simulink model "gm_dadda_mult"  (R2015a)
settings: Solver=ode45  StartTime=0.0  StopTime=10.0  RelTol=1e-3
settings Model: Creator=citdmath  LastModifiedBy=citdmath
settings OptimizationCC: BlockReduction=off  ConditionallyExecuteInputs=off
settings DebuggingCC: InheritedTsInSrcMsg=none

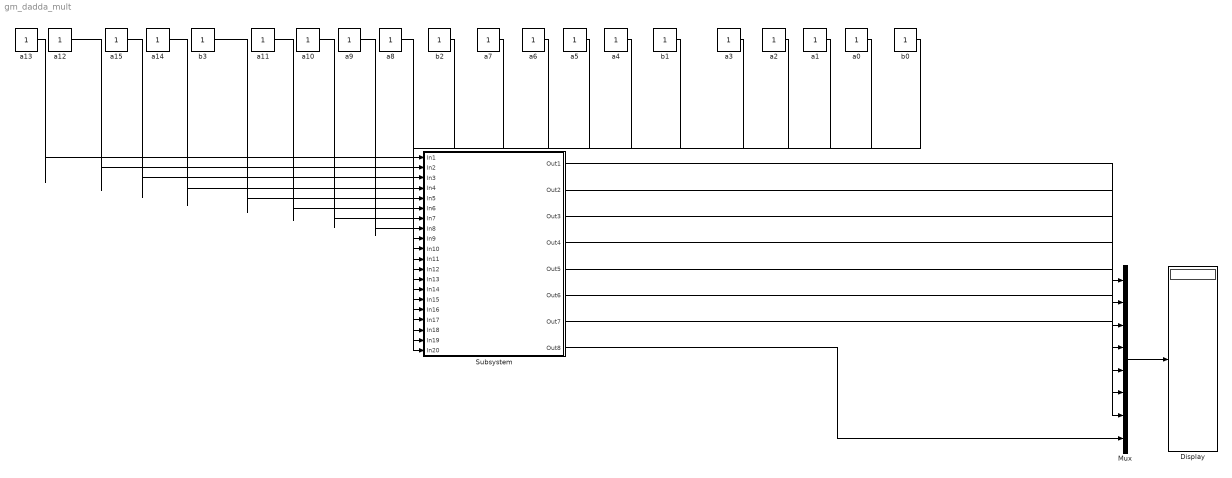
== system gm_dadda_mult ==
  Display : Display
  Mux : Mux  Inputs=8
  Subsystem : Subsystem
  a{0..15} (16 alike) : Constant
  b{0..3} (4 alike) : Constant
  wires:
  Subsystem/8(Out8) -> Mux/8
  Subsystem/7(Out7) -> Mux/7
  Subsystem/6(Out6) -> Mux/6
  Subsystem/5(Out5) -> Mux/5
  Subsystem/4(Out4) -> Mux/4
  Subsystem/3(Out3) -> Mux/3
  Subsystem/2(Out2) -> Mux/2
  Subsystem/1(Out1) -> Mux/1
  b0/1 -> Subsystem/20(In20)
  a0/1 -> Subsystem/19(In19)
  a1/1 -> Subsystem/18(In18)
  a2/1 -> Subsystem/17(In17)
  a3/1 -> Subsystem/16(In16)
  b1/1 -> Subsystem/15(In15)
  a4/1 -> Subsystem/14(In14)
  a5/1 -> Subsystem/13(In13)
  a6/1 -> Subsystem/12(In12)
  a7/1 -> Subsystem/11(In11)
  b2/1 -> Subsystem/10(In10)
  a8/1 -> Subsystem/9(In9)
  a9/1 -> Subsystem/8(In8)
  a10/1 -> Subsystem/7(In7)
  a11/1 -> Subsystem/6(In6)
  b3/1 -> Subsystem/5(In5)
  a14/1 -> Subsystem/4(In4)
  a15/1 -> Subsystem/3(In3)
  a12/1 -> Subsystem/2(In2)
  a13/1 -> Subsystem/1(In1)
  Mux/1 -> Display/1

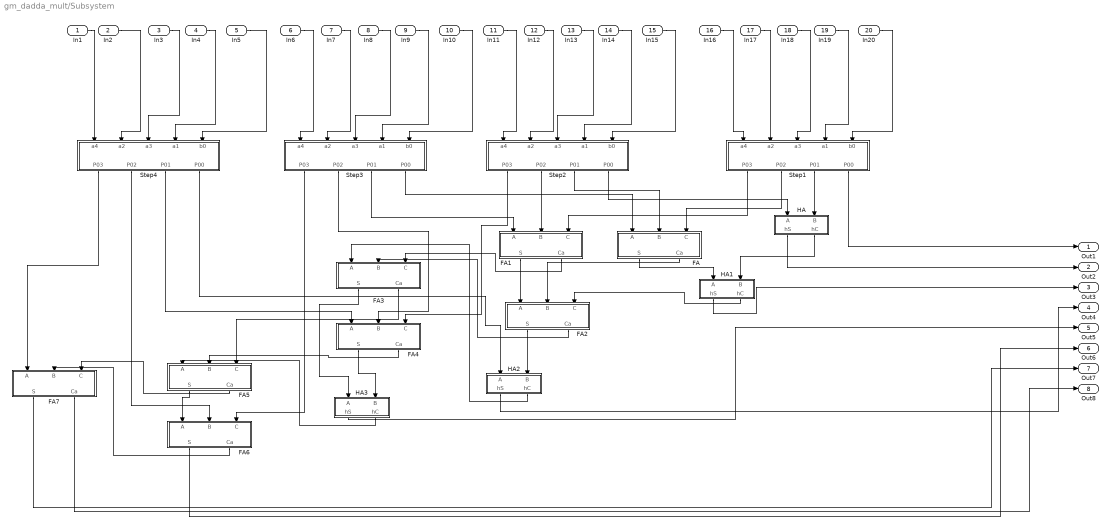
== system gm_dadda_mult/Subsystem ==
  In1 : Inport
  In2 : Inport  Port=2
  In3 : Inport  Port=3
  In4 : Inport  Port=4
  In5 : Inport  Port=5
  In6 : Inport  Port=6
  In7 : Inport  Port=7
  In8 : Inport  Port=8
  In9 : Inport  Port=9
  In10 : Inport  Port=10
  In11 : Inport  Port=11
  In12 : Inport  Port=12
  In13 : Inport  Port=13
  In14 : Inport  Port=14
  In15 : Inport  Port=15
  In16 : Inport  Port=16
  In17 : Inport  Port=17
  In18 : Inport  Port=18
  In19 : Inport  Port=19
  In20 : Inport  Port=20
  FA : Subsystem
  FA1 : Subsystem
  FA2 : Subsystem
  FA3 : Subsystem
  FA4 : Subsystem
  FA5 : Subsystem
  FA6 : Subsystem
  FA7 : Subsystem
  HA : Subsystem
  HA1 : Subsystem
  HA2 : Subsystem
  HA3 : Subsystem
  Step1 : Subsystem
  Step2 : Subsystem
  Step3 : Subsystem
  Step4 : Subsystem
  Out1 : Outport
  Out2 : Outport  Port=2
  Out3 : Outport  Port=3
  Out4 : Outport  Port=4
  Out5 : Outport  Port=5
  Out6 : Outport  Port=6
  Out7 : Outport  Port=7
  Out8 : Outport  Port=8
  wires:
  FA/2(Ca) -> FA2/2(B)
  Step3/3(P01) -> FA1/1(A)
  FA5/1(S) -> FA6/1(A)
  FA2/1(S) -> HA2/2(B)
  FA2/2(Ca) -> FA3/2(B)
  HA2/1(hS) -> Out4/1
  Step2/2(P02) -> FA1/2(B)
  Step2/1(P03) -> FA4/3(C)
  FA1/2(Ca) -> FA3/3(C)
  FA1/1(S) -> FA2/1(A)
  HA3/2(hC) -> FA5/1(A)
  FA5/2(Ca) -> FA7/3(C)
  FA4/1(S) -> HA3/2(B)
  FA7/2(Ca) -> Out8/1
  FA3/2(Ca) -> FA5/3(C)
  FA3/1(S) -> HA3/1(A)
  Step1/1(P03) -> FA1/3(C)
  Step4/4(P00) -> HA2/1(A)
  HA1/1(hS) -> Out3/1
  HA1/2(hC) -> FA2/3(C)
  FA/1(S) -> HA1/1(A)
  HA3/1(hS) -> Out5/1
  FA7/1(S) -> Out7/1
  HA/2(hC) -> HA1/2(B)
  Step4/2(P02) -> FA6/2(B)
  Step3/2(P02) -> FA4/2(B)
  Step1/4(P00) -> Out1/1
  FA4/2(Ca) -> FA5/2(B)
  FA6/2(Ca) -> FA7/2(B)
  Step2/4(P00) -> HA/1(A)
  Step3/1(P03) -> FA6/3(C)
  HA/1(hS) -> Out2/1
  Step4/3(P01) -> FA4/1(A)
  Step3/4(P00) -> FA/1(A)
  In20/1 -> Step1/5(b0)
  In1/1 -> Step4/1(a4)
  In5/1 -> Step4/5(b0)
  Step1/3(P01) -> HA/2(B)
  In2/1 -> Step4/2(a2)
  In4/1 -> Step4/4(a1)
  In3/1 -> Step4/3(a3)
  In16/1 -> Step1/1(a4)
  Step4/1(P03) -> FA7/1(A)
  In9/1 -> Step3/4(a1)
  In7/1 -> Step3/2(a2)
  In6/1 -> Step3/1(a4)
  In8/1 -> Step3/3(a3)
  In10/1 -> Step3/5(b0)
  FA6/1(S) -> Out6/1
  In18/1 -> Step1/3(a3)
  In12/1 -> Step2/2(a2)
  In13/1 -> Step2/3(a3)
  In14/1 -> Step2/4(a1)
  In15/1 -> Step2/5(b0)
  In11/1 -> Step2/1(a4)
  In17/1 -> Step1/2(a2)
  HA2/2(hC) -> FA3/1(A)
  Step2/3(P01) -> FA/2(B)
  Step1/2(P02) -> FA/3(C)
  In19/1 -> Step1/4(a1)

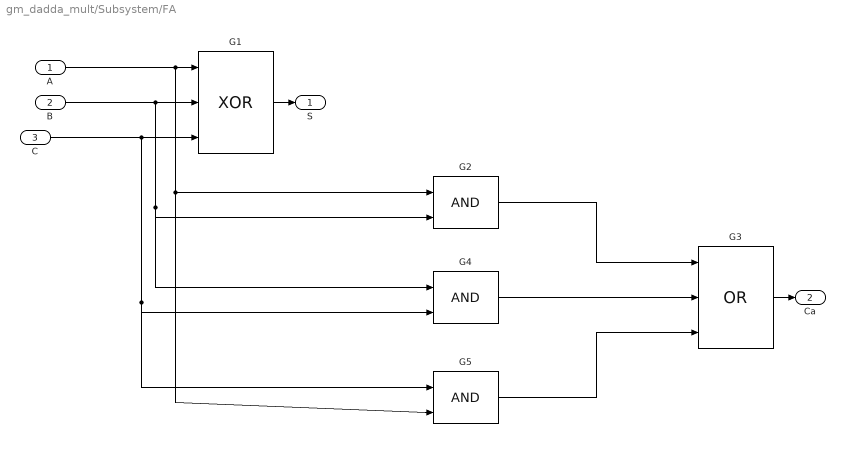
== system gm_dadda_mult/Subsystem/FA ==
  A : Inport
  B : Inport  Port=2
  C : Inport  Port=3
  G1 : Logic  Operator=XOR  Inputs=3  IconShape=distinctive  AllPortsSameDT=off  OutDataTypeStr=boolean
  G2 : Logic  IconShape=distinctive  AllPortsSameDT=off  OutDataTypeStr=boolean
  G3 : Logic  Operator=OR  Inputs=3  IconShape=distinctive  AllPortsSameDT=off  OutDataTypeStr=boolean
  G4 : Logic  IconShape=distinctive  AllPortsSameDT=off  OutDataTypeStr=boolean
  G5 : Logic  IconShape=distinctive  AllPortsSameDT=off  OutDataTypeStr=boolean
  S : Outport
  Ca : Outport  Port=2
  wires:
  G1/1 -> S/1
  G3/1 -> Ca/1
  B/1 -> G1/2, G2/2, G4/1
  G4/1 -> G3/2
  A/1 -> G1/1, G2/1, G5/2
  G2/1 -> G3/1
  C/1 -> G1/3, G4/2, G5/1
  G5/1 -> G3/3

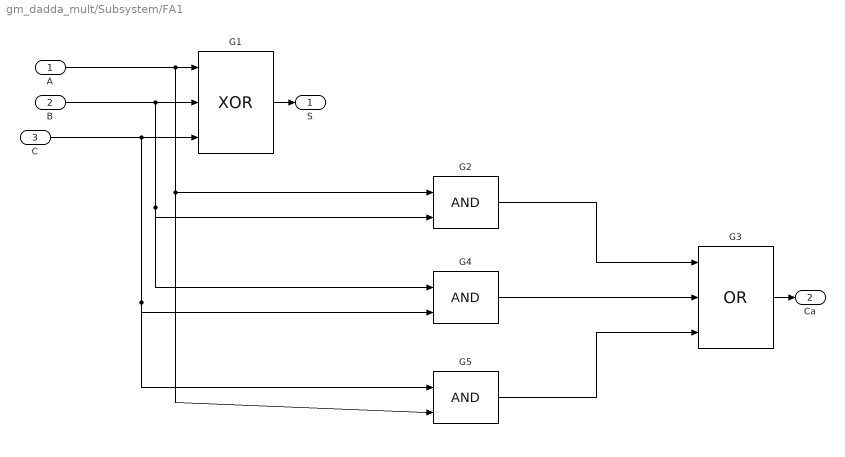
== system gm_dadda_mult/Subsystem/FA1 ==
  A : Inport
  B : Inport  Port=2
  C : Inport  Port=3
  G1 : Logic  Operator=XOR  Inputs=3  IconShape=distinctive  AllPortsSameDT=off  OutDataTypeStr=boolean
  G2 : Logic  IconShape=distinctive  AllPortsSameDT=off  OutDataTypeStr=boolean
  G3 : Logic  Operator=OR  Inputs=3  IconShape=distinctive  AllPortsSameDT=off  OutDataTypeStr=boolean
  G4 : Logic  IconShape=distinctive  AllPortsSameDT=off  OutDataTypeStr=boolean
  G5 : Logic  IconShape=distinctive  AllPortsSameDT=off  OutDataTypeStr=boolean
  S : Outport
  Ca : Outport  Port=2
  wires:
  G5/1 -> G3/3
  C/1 -> G5/1, G4/2, G1/3
  G2/1 -> G3/1
  A/1 -> G5/2, G2/1, G1/1
  G4/1 -> G3/2
  B/1 -> G4/1, G2/2, G1/2
  G3/1 -> Ca/1
  G1/1 -> S/1

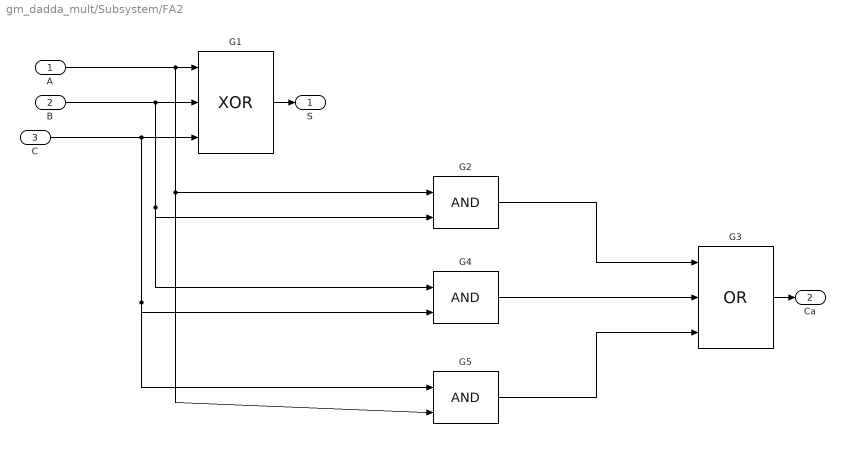
== system gm_dadda_mult/Subsystem/FA2 ==
  A : Inport
  B : Inport  Port=2
  C : Inport  Port=3
  G1 : Logic  Operator=XOR  Inputs=3  IconShape=distinctive  AllPortsSameDT=off  OutDataTypeStr=boolean
  G2 : Logic  IconShape=distinctive  AllPortsSameDT=off  OutDataTypeStr=boolean
  G3 : Logic  Operator=OR  Inputs=3  IconShape=distinctive  AllPortsSameDT=off  OutDataTypeStr=boolean
  G4 : Logic  IconShape=distinctive  AllPortsSameDT=off  OutDataTypeStr=boolean
  G5 : Logic  IconShape=distinctive  AllPortsSameDT=off  OutDataTypeStr=boolean
  S : Outport
  Ca : Outport  Port=2
  wires:
  G1/1 -> S/1
  G3/1 -> Ca/1
  B/1 -> G1/2, G2/2, G4/1
  G4/1 -> G3/2
  A/1 -> G1/1, G2/1, G5/2
  G2/1 -> G3/1
  C/1 -> G1/3, G4/2, G5/1
  G5/1 -> G3/3

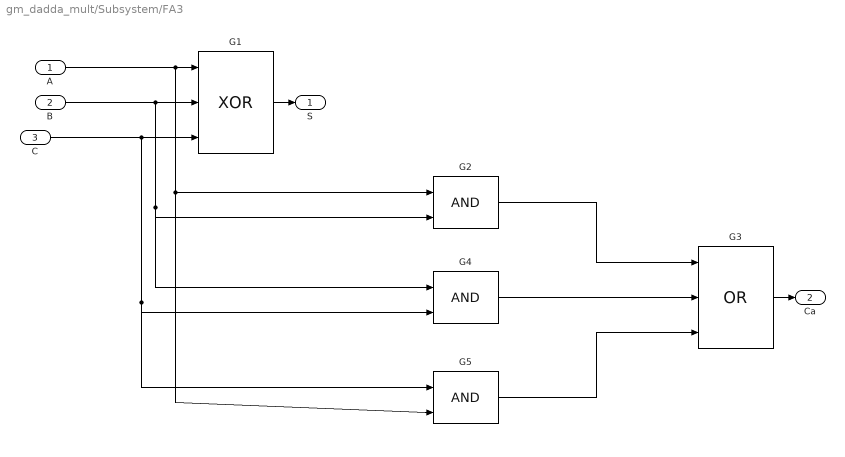
== system gm_dadda_mult/Subsystem/FA3 ==
  A : Inport
  B : Inport  Port=2
  C : Inport  Port=3
  G1 : Logic  Operator=XOR  Inputs=3  IconShape=distinctive  AllPortsSameDT=off  OutDataTypeStr=boolean
  G2 : Logic  IconShape=distinctive  AllPortsSameDT=off  OutDataTypeStr=boolean
  G3 : Logic  Operator=OR  Inputs=3  IconShape=distinctive  AllPortsSameDT=off  OutDataTypeStr=boolean
  G4 : Logic  IconShape=distinctive  AllPortsSameDT=off  OutDataTypeStr=boolean
  G5 : Logic  IconShape=distinctive  AllPortsSameDT=off  OutDataTypeStr=boolean
  S : Outport
  Ca : Outport  Port=2
  wires:
  G1/1 -> S/1
  G3/1 -> Ca/1
  B/1 -> G1/2, G2/2, G4/1
  G4/1 -> G3/2
  A/1 -> G1/1, G2/1, G5/2
  G2/1 -> G3/1
  C/1 -> G1/3, G4/2, G5/1
  G5/1 -> G3/3

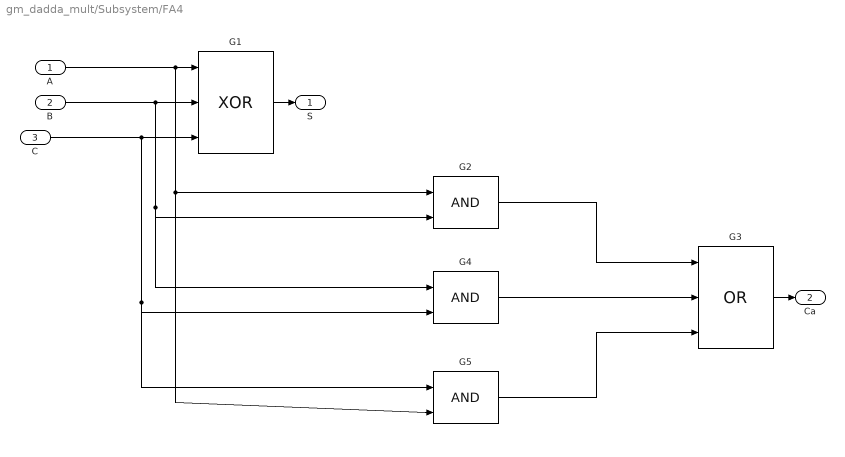
== system gm_dadda_mult/Subsystem/FA4 ==
  A : Inport
  B : Inport  Port=2
  C : Inport  Port=3
  G1 : Logic  Operator=XOR  Inputs=3  IconShape=distinctive  AllPortsSameDT=off  OutDataTypeStr=boolean
  G2 : Logic  IconShape=distinctive  AllPortsSameDT=off  OutDataTypeStr=boolean
  G3 : Logic  Operator=OR  Inputs=3  IconShape=distinctive  AllPortsSameDT=off  OutDataTypeStr=boolean
  G4 : Logic  IconShape=distinctive  AllPortsSameDT=off  OutDataTypeStr=boolean
  G5 : Logic  IconShape=distinctive  AllPortsSameDT=off  OutDataTypeStr=boolean
  S : Outport
  Ca : Outport  Port=2
  wires:
  G5/1 -> G3/3
  C/1 -> G5/1, G4/2, G1/3
  G2/1 -> G3/1
  A/1 -> G5/2, G2/1, G1/1
  G4/1 -> G3/2
  B/1 -> G4/1, G2/2, G1/2
  G3/1 -> Ca/1
  G1/1 -> S/1

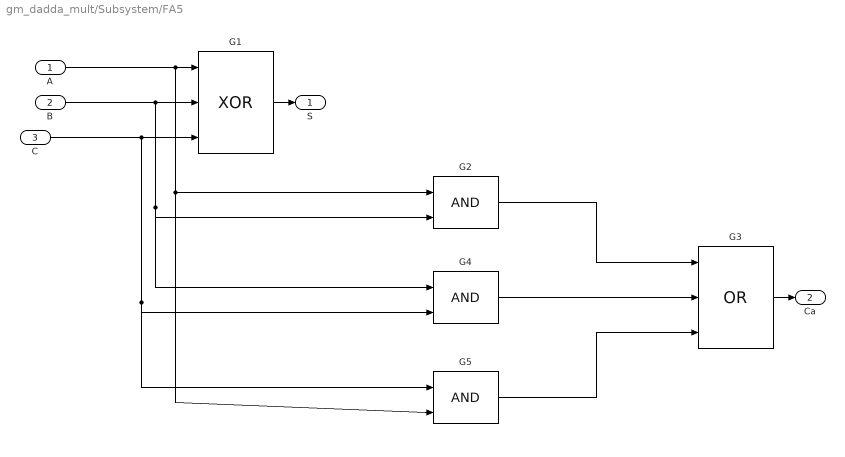
== system gm_dadda_mult/Subsystem/FA5 ==
  A : Inport
  B : Inport  Port=2
  C : Inport  Port=3
  G1 : Logic  Operator=XOR  Inputs=3  IconShape=distinctive  AllPortsSameDT=off  OutDataTypeStr=boolean
  G2 : Logic  IconShape=distinctive  AllPortsSameDT=off  OutDataTypeStr=boolean
  G3 : Logic  Operator=OR  Inputs=3  IconShape=distinctive  AllPortsSameDT=off  OutDataTypeStr=boolean
  G4 : Logic  IconShape=distinctive  AllPortsSameDT=off  OutDataTypeStr=boolean
  G5 : Logic  IconShape=distinctive  AllPortsSameDT=off  OutDataTypeStr=boolean
  S : Outport
  Ca : Outport  Port=2
  wires:
  G5/1 -> G3/3
  C/1 -> G5/1, G4/2, G1/3
  G2/1 -> G3/1
  A/1 -> G5/2, G2/1, G1/1
  G4/1 -> G3/2
  B/1 -> G4/1, G2/2, G1/2
  G3/1 -> Ca/1
  G1/1 -> S/1

== system gm_dadda_mult/Subsystem/FA6 ==
  A : Inport
  B : Inport  Port=2
  C : Inport  Port=3
  G1 : Logic  Operator=XOR  Inputs=3  IconShape=distinctive  AllPortsSameDT=off  OutDataTypeStr=boolean
  G2 : Logic  IconShape=distinctive  AllPortsSameDT=off  OutDataTypeStr=boolean
  G3 : Logic  Operator=OR  Inputs=3  IconShape=distinctive  AllPortsSameDT=off  OutDataTypeStr=boolean
  G4 : Logic  IconShape=distinctive  AllPortsSameDT=off  OutDataTypeStr=boolean
  G5 : Logic  IconShape=distinctive  AllPortsSameDT=off  OutDataTypeStr=boolean
  S : Outport
  Ca : Outport  Port=2
  wires:
  G1/1 -> S/1
  G3/1 -> Ca/1
  B/1 -> G1/2, G2/2, G4/1
  G4/1 -> G3/2
  A/1 -> G1/1, G2/1, G5/2
  G2/1 -> G3/1
  C/1 -> G1/3, G4/2, G5/1
  G5/1 -> G3/3

== system gm_dadda_mult/Subsystem/FA7 ==
  A : Inport
  B : Inport  Port=2
  C : Inport  Port=3
  G1 : Logic  Operator=XOR  Inputs=3  IconShape=distinctive  AllPortsSameDT=off  OutDataTypeStr=boolean
  G2 : Logic  IconShape=distinctive  AllPortsSameDT=off  OutDataTypeStr=boolean
  G3 : Logic  Operator=OR  Inputs=3  IconShape=distinctive  AllPortsSameDT=off  OutDataTypeStr=boolean
  G4 : Logic  IconShape=distinctive  AllPortsSameDT=off  OutDataTypeStr=boolean
  G5 : Logic  IconShape=distinctive  AllPortsSameDT=off  OutDataTypeStr=boolean
  S : Outport
  Ca : Outport  Port=2
  wires:
  G1/1 -> S/1
  G3/1 -> Ca/1
  B/1 -> G1/2, G2/2, G4/1
  G4/1 -> G3/2
  A/1 -> G1/1, G2/1, G5/2
  G2/1 -> G3/1
  C/1 -> G1/3, G4/2, G5/1
  G5/1 -> G3/3

== system gm_dadda_mult/Subsystem/HA ==
  A : Inport
  B : Inport  Port=2
  G1 : Logic  Operator=XOR  IconShape=distinctive  AllPortsSameDT=off  OutDataTypeStr=boolean
  G2 : Logic  IconShape=distinctive  AllPortsSameDT=off  OutDataTypeStr=boolean
  hS : Outport
  hC : Outport  Port=2
  wires:
  G1/1 -> hS/1  "hS"
  G2/1 -> hC/1  "hC"
  B/1 -> G2/2, G1/2
  A/1 -> G1/1, G2/1

== system gm_dadda_mult/Subsystem/HA1 ==
  A : Inport
  B : Inport  Port=2
  G1 : Logic  Operator=XOR  IconShape=distinctive  AllPortsSameDT=off  OutDataTypeStr=boolean
  G2 : Logic  IconShape=distinctive  AllPortsSameDT=off  OutDataTypeStr=boolean
  hS : Outport
  hC : Outport  Port=2
  wires:
  A/1 -> G2/1, G1/1
  B/1 -> G1/2, G2/2
  G2/1 -> hC/1  "hC"
  G1/1 -> hS/1  "hS"

== system gm_dadda_mult/Subsystem/HA2 ==
  A : Inport
  B : Inport  Port=2
  G1 : Logic  Operator=XOR  IconShape=distinctive  AllPortsSameDT=off  OutDataTypeStr=boolean
  G2 : Logic  IconShape=distinctive  AllPortsSameDT=off  OutDataTypeStr=boolean
  hS : Outport
  hC : Outport  Port=2
  wires:
  G1/1 -> hS/1  "hS"
  G2/1 -> hC/1  "hC"
  B/1 -> G2/2, G1/2
  A/1 -> G1/1, G2/1

== system gm_dadda_mult/Subsystem/HA3 ==
  A : Inport
  B : Inport  Port=2
  G1 : Logic  Operator=XOR  IconShape=distinctive  AllPortsSameDT=off  OutDataTypeStr=boolean
  G2 : Logic  IconShape=distinctive  AllPortsSameDT=off  OutDataTypeStr=boolean
  hS : Outport
  hC : Outport  Port=2
  wires:
  A/1 -> G2/1, G1/1
  B/1 -> G1/2, G2/2
  G2/1 -> hC/1  "hC"
  G1/1 -> hS/1  "hS"

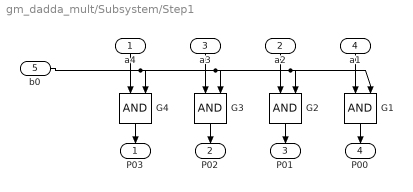
== system gm_dadda_mult/Subsystem/Step1 ==
  a4 : Inport
  a2 : Inport  Port=2
  a3 : Inport  Port=3
  a1 : Inport  Port=4
  b0 : Inport  Port=5
  G{1..4} (4 alike) : Logic  IconShape=distinctive  AllPortsSameDT=off  OutDataTypeStr=boolean
  P03 : Outport
  P02 : Outport  Port=2
  P01 : Outport  Port=3
  P00 : Outport  Port=4
  wires:
  G3/1 -> P02/1
  G2/1 -> P01/1
  G1/1 -> P00/1
  G4/1 -> P03/1
  a2/1 -> G2/1
  a4/1 -> G4/1
  b0/1 -> G4/2, G3/2, G2/2, G1/2
  a1/1 -> G1/1
  a3/1 -> G3/1

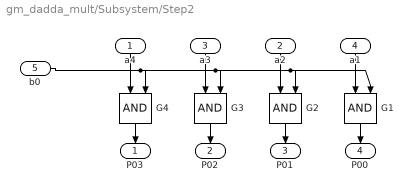
== system gm_dadda_mult/Subsystem/Step2 ==
  a4 : Inport
  a2 : Inport  Port=2
  a3 : Inport  Port=3
  a1 : Inport  Port=4
  b0 : Inport  Port=5
  G{1..4} (4 alike) : Logic  IconShape=distinctive  AllPortsSameDT=off  OutDataTypeStr=boolean
  P03 : Outport
  P02 : Outport  Port=2
  P01 : Outport  Port=3
  P00 : Outport  Port=4
  wires:
  a3/1 -> G3/1
  a1/1 -> G1/1
  b0/1 -> G1/2, G2/2, G3/2, G4/2
  a4/1 -> G4/1
  a2/1 -> G2/1
  G4/1 -> P03/1
  G1/1 -> P00/1
  G2/1 -> P01/1
  G3/1 -> P02/1

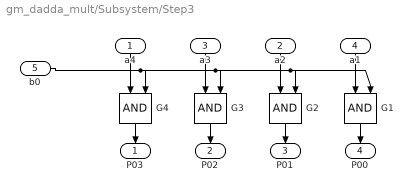
== system gm_dadda_mult/Subsystem/Step3 ==
  a4 : Inport
  a2 : Inport  Port=2
  a3 : Inport  Port=3
  a1 : Inport  Port=4
  b0 : Inport  Port=5
  G{1..4} (4 alike) : Logic  IconShape=distinctive  AllPortsSameDT=off  OutDataTypeStr=boolean
  P03 : Outport
  P02 : Outport  Port=2
  P01 : Outport  Port=3
  P00 : Outport  Port=4
  wires:
  G3/1 -> P02/1
  G2/1 -> P01/1
  G1/1 -> P00/1
  G4/1 -> P03/1
  a2/1 -> G2/1
  a4/1 -> G4/1
  b0/1 -> G4/2, G3/2, G2/2, G1/2
  a1/1 -> G1/1
  a3/1 -> G3/1

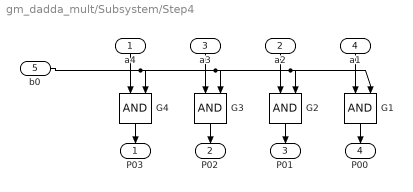
== system gm_dadda_mult/Subsystem/Step4 ==
  a4 : Inport
  a2 : Inport  Port=2
  a3 : Inport  Port=3
  a1 : Inport  Port=4
  b0 : Inport  Port=5
  G{1..4} (4 alike) : Logic  IconShape=distinctive  AllPortsSameDT=off  OutDataTypeStr=boolean
  P03 : Outport
  P02 : Outport  Port=2
  P01 : Outport  Port=3
  P00 : Outport  Port=4
  wires:
  a3/1 -> G3/1
  a1/1 -> G1/1
  b0/1 -> G1/2, G2/2, G3/2, G4/2
  a4/1 -> G4/1
  a2/1 -> G2/1
  G4/1 -> P03/1
  G1/1 -> P00/1
  G2/1 -> P01/1
  G3/1 -> P02/1
